simulink model "my_converter"  (R2024a)
settings: Solver=ode45  StartTime=0.0  StopTime=1  RelTol=1e-3
libraries: spsMosfetLib x10, spsSeriesRLCBranchLib x7, spsCurrentMeasurementLib x1, spsPVArrayLib x1, spsPWMGeneratorDCDCLib x1, spsVoltageMeasurementLib x1, sps_lib x1
settings Model: Creator=Administrator  LastModifiedBy=ZTH
settings DebuggingCC: AlgebraicLoopMsg=none
settings RTWCC: GPUComputeCapability=3.5

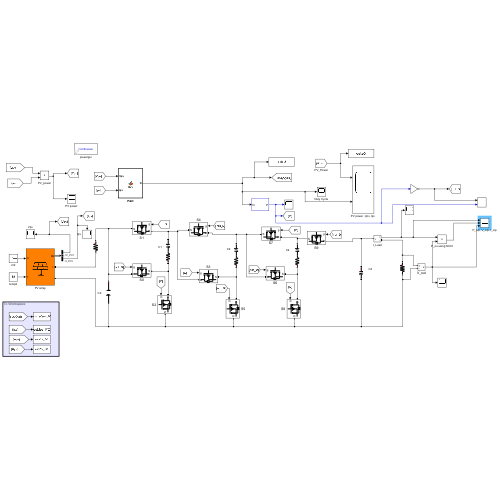
[thumbnail: Simulink's stored preview of the top-level diagram]
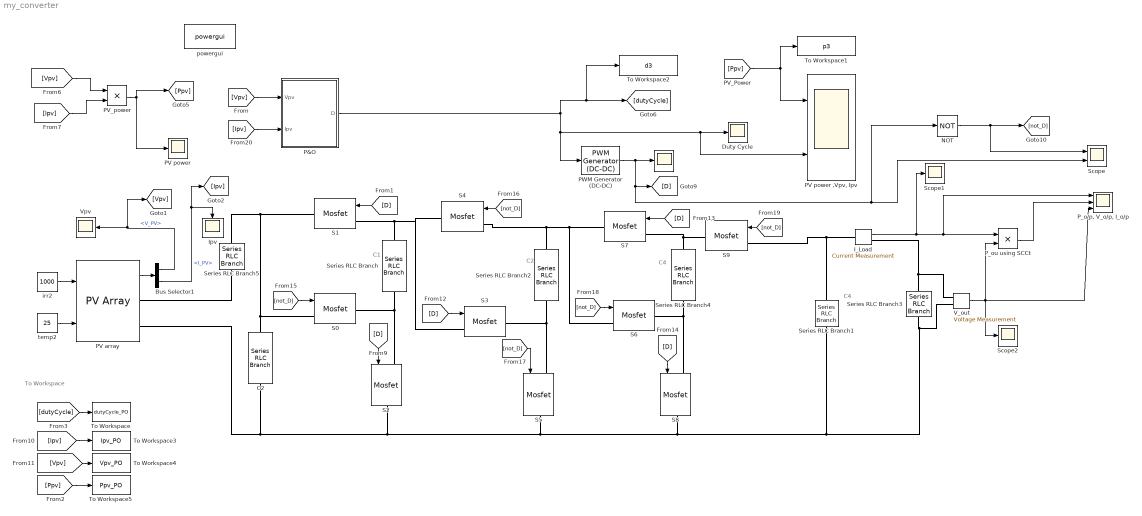
== system my_converter ==
  note: C4
  note: C4
  note: C2
  note: C1
  note: To Workspace
  " " : Scope
  Bus Selector1 : BusSelector  OutputSignals=V_PV,I_PV
  C2 : spsSeriesRLCBranchLib/Series RLC Branch  LConnTagsString=__new0  RConnTagsString=__new0  BranchType=C  Resistance=0.0001  Inductance=1e-3  SetiL0=off  InitialCurrent=0  Capacitance=1e-2  Setx0=on  InitialVoltage=0  Measurements=None
  Duty Cycle : Scope
  I_Load : spsCurrentMeasurementLib/Current Measurement  PhasorSimulation=off  OutputType=Magnitude  PSBequivalent=0
  Ipv : Scope
  NOT : Logic  Operator=NOT  IconShape=distinctive  AllPortsSameDT=off  OutDataTypeStr=boolean
  P&O : MATLAB Function  TreatAsAtomicUnit=on
  PV array : spsPVArrayLib/PV Array  Npar=3  Nser=3  PlotType=array @ 1000 W/m2 & specified temperatures  S_vec="[ 1000  500  100 ]"  Temp_C_vec="[ 45 25  ]"  ModuleName=User-defined  PlotWhenSelected=off  Pm=334.905  Ncell=80  Voc=49.9  Isc=9  Vm=41.5  Im=8.07  beta_Voc_pc=-0.36  alpha_Isc_pc=0.09  beta_Voc=-0.17964  alpha_Isc=0.0081  IL=9.0297  I0=3.1312e-10  nI=1.0111  Rsh=77.6407  Rs=0.25633  RobustModel=off  RobustCellTemperature=313.3991  BAL=on  Tc=1e-6  Tfilter=5e-5
  PV power : Scope
  "PV power ,Vpv, Ipv " : Scope  NumInputPorts=2
  PV_power : Product
  PWM Generator (DC-DC) : spsPWMGeneratorDCDCLib/PWM Generator (DC-DC)  Fsw=5e3  Ts=0
  "P_o/p, V_o/p, I_o/p" : Scope  NumInputPorts=3
  P_ou using SCCt : Product
  S{0..9} (10 alike) : spsMosfetLib/Mosfet  Ron=1e-3  Lon=0  Rd=1e-3  Vfd=0  IC=0  Rs=inf  Cs=inf  Measurements=off
  Scope : Scope  NumInputPorts=2
  Scope1 : Scope
  Scope2 : Scope
  Series RLC Branch : spsSeriesRLCBranchLib/Series RLC Branch  LConnTagsString=__new0  RConnTagsString=__new0  BranchType=RC  Resistance=0.1  Inductance=1e-3  SetiL0=off  InitialCurrent=0  Capacitance=2e-3  Setx0=off  InitialVoltage=0  Measurements=None
  Series RLC Branch1 : spsSeriesRLCBranchLib/Series RLC Branch  LConnTagsString=__new0  RConnTagsString=__new0  BranchType=C  Resistance=1e-4  Inductance=200e-6  SetiL0=off  InitialCurrent=0  Capacitance=2e-3  Setx0=off  InitialVoltage=40  Measurements=None
  Series RLC Branch2 : spsSeriesRLCBranchLib/Series RLC Branch  LConnTagsString=__new0  RConnTagsString=__new0  BranchType=RC  Resistance=0.1  Inductance=1e-3  SetiL0=off  InitialCurrent=0  Capacitance=2e-3  Setx0=off  InitialVoltage=0  Measurements=None
  Series RLC Branch3 : spsSeriesRLCBranchLib/Series RLC Branch  LConnTagsString=__new0  RConnTagsString=__new0  BranchType=R  Resistance=130  Inductance=200e-6  SetiL0=off  InitialCurrent=0  Capacitance=1000e-6  Setx0=off  InitialVoltage=40  Measurements=None
  Series RLC Branch4 : spsSeriesRLCBranchLib/Series RLC Branch  LConnTagsString=__new0  RConnTagsString=__new0  BranchType=RC  Resistance=0.1  Inductance=1e-3  SetiL0=off  InitialCurrent=0  Capacitance=2e-3  Setx0=off  InitialVoltage=0  Measurements=None
  Series RLC Branch5 : spsSeriesRLCBranchLib/Series RLC Branch  LConnTagsString=__new0  RConnTagsString=__new0  BranchType=R  Resistance=0.1  Inductance=200e-6  SetiL0=off  InitialCurrent=0  Capacitance=1000e-6  Setx0=off  InitialVoltage=40  Measurements=None
  To Workspace : ToWorkspace  VariableName=dutyCycle_PO  SampleTime=-1
  To Workspace1 : ToWorkspace  VariableName=p3  SaveFormat=Timeseries  SampleTime=-1
  To Workspace2 : ToWorkspace  VariableName=d3  SaveFormat=Timeseries  SampleTime=-1
  To Workspace3 : ToWorkspace  VariableName=Ipv_PO  SampleTime=-1
  To Workspace4 : ToWorkspace  VariableName=Vpv_PO  SampleTime=-1
  To Workspace5 : ToWorkspace  VariableName=Ppv_PO  SampleTime=-1
  V_out : spsVoltageMeasurementLib/Voltage Measurement  PhasorSimulation=off  OutputType=Magnitude  PSBequivalent=0
  Vpv : Scope
  irr2 : Constant  Value=1000
  powergui : sps_lib/powergui  Priority=1  SimulationMode=Continuous  SampleTime=50e-6  frequency=60  Iterations=50  frequencyindice=0  Pbase=100e6  ErrMax=1e-4  UnitsV=kV  UnitsW=MW  buscounter=0  FunctionMessages=off  echomessages=off  EnableUseOfTLC=off  CurrentSourceSwitches=off  DisableSnubberDevices=off  DisableRonSwitches=off  DisableVfSwitches=off  DisplayEquations=off  AutomaticDiscreteSolvers=off  SolverType=Tustin/Backward Euler (TBE)  Interpol=off  ExternalGateDelay=off  methode=off  Ts=100  x0status=blocks  SPID=on  SwTol=0  HookPort=off  NonlinearTolerance=1e-4  nMaxIteration=100  ContinueOnMaxIteration=off  RestoreLinks=warning  ResistiveCurrentMeasurement=off  Frange=[0:2:500]  Ylog=off  Xlog=on  ShowGrid=off  save=off  variable=ZData  structure=0  ZoomFFT=off  StartTime=0.0  cycles=1  DisplayStyle=1  fundamental=60  FreqAxis=off  MaxFrequency=1000  frequencyindicesteady=1  RmsSteady=1  display=off
  temp2 : Constant  Value=25
  wires:
  [Ppv] -> "PV power ,Vpv, Ipv "/1, To Workspace1/1
  V_out/1 -> Scope2/1, P_ou using SCCt/2, "P_o/p, V_o/p, I_o/p"/3
  temp2/1 -> PV array/2
  [dutyCycle] -> To Workspace/1
  [Ipv] -> PV_power/2
  [Vpv] -> PV_power/1
  irr2/1 -> PV array/1
  I_Load/1 -> Scope1/1, "P_o/p, V_o/p, I_o/p"/1, P_ou using SCCt/1
  PV array/1 -> Bus Selector1/1
  [Ipv] -> To Workspace3/1
  PV_power/1 -> PV power/1, [Ppv]
  [Vpv] -> To Workspace4/1
  [Ppv] -> To Workspace5/1
  P&O/1(D) -> PWM Generator (DC-DC)/1, "PV power ,Vpv, Ipv "/2, Duty Cycle/1, [dutyCycle], To Workspace2/1
  PWM Generator (DC-DC)/1 -> Scope/2, NOT/1, [D], " "/1
  [D] -> S1/1
  [D] -> S3/1
  [D] -> S7/1
  NOT/1 -> Scope/1, [not_D]
  [not_D] -> S0/1
  [not_D] -> S4/1
  [not_D] -> S6/1
  [D] -> S2/1
  [D] -> S8/1
  [not_D] -> S9/1
  Bus Selector1/1 -> [Vpv], Vpv/1  "<V_PV>"
  Bus Selector1/2 -> [Ipv], Ipv/1  "<I_PV>"
  [not_D] -> S5/1
  [Ipv] -> P&O/2(Ipv)
  [Vpv] -> P&O/1(Vpv)
  P_ou using SCCt/1 -> "P_o/p, V_o/p, I_o/p"/2
  connections:
  C2/LConn1 -- S0/LConn1 -- Series RLC Branch5/LConn1 -- S1/RConn1
  Series RLC Branch/RConn1 -- S4/RConn1 -- S3/LConn1 -- S1/LConn1
  Series RLC Branch3/LConn1 -- I_Load/RConn1 -- V_out/LConn1
  Series RLC Branch3/RConn1 -- V_out/LConn2 -- Series RLC Branch1/RConn1 -- S8/RConn1 -- S5/RConn1 -- S2/RConn1 -- PV array/RConn2 -- C2/RConn1
  Series RLC Branch/LConn1 -- S2/LConn1 -- S0/RConn1
  S5/LConn1 -- S3/RConn1 -- Series RLC Branch2/LConn1
  S4/LConn1 -- Series RLC Branch2/RConn1 -- S6/LConn1 -- S7/RConn1
  Series RLC Branch4/LConn1 -- S6/RConn1 -- S8/LConn1
  Series RLC Branch4/RConn1 -- S9/RConn1 -- S7/LConn1
  I_Load/LConn1 -- Series RLC Branch1/LConn1 -- S9/LConn1
  PV array/RConn1 -- Series RLC Branch5/RConn1

== matlab function my_converter/P&O ==
  settings: updateMethod=DISCRETE  sampleTime=1e-4
  data: Vpv input; D output; Ipv input
function D = PO(Vpv,Ipv)
 Dmax=0.9;
 Dmin=0.1;
 Dinit=0.9;
 deltaD=2e-3;
 persistent Dpre Ppre Vpre;
 
 %first run
     if isempty(Dpre)
         Dpre=Dinit;
         Vpre=0;
         Ppre=0;
     end
 Ppv=Vpv*Ipv;
 dp=Ppv-Ppre;
 dv=Vpv-Vpre;
 
     if dp~=0 
             if(dp>0)
                     if(dv<0)
                         D=Dpre+deltaD;
                     else
                         D=Dpre-deltaD;
                     end     
             else                   
                     if(dv<0)
                         D=Dpre-deltaD;
                     else
                         D=Dpre+deltaD;
                     end
             end   
    else
          D=Dpre;
    end
    
    if D>=Dmax || D <= Dmin
        D=Dpre;
    end
    
    Ppre=Ppv;
    Vpre=Vpv;
    Dpre=D;
end
